simulink library "speedgoatlib"  (Simulink 7.6)
settings: Solver=ode45  StartTime=0.0  StopTime=10.0  RelTol=1e-3
undefined symbols (not defined in the file): m_XR17D15x, mmodemcontrol, standard
libraries: speedgoatlib x176, xpcseriallib x84, xpclib x4, simulink x4
(part 3 of 4)

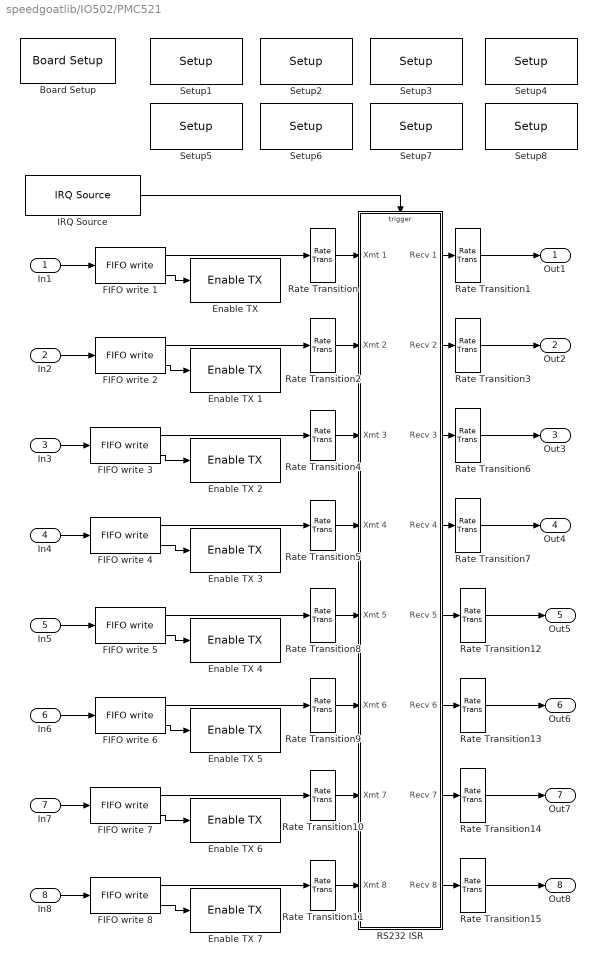
== system speedgoatlib/IO502/PMC521 ==
  In1 : Inport
  In2 : Inport  Port=2
  In3 : Inport  Port=3
  In4 : Inport  Port=4
  In5 : Inport  Port=5
  In6 : Inport  Port=6
  In7 : Inport  Port=7
  In8 : Inport  Port=8
  Board Setup : speedgoatlib/IO502/Acromag PMC521 Internal blocks/Board Setup  reffreq=14745600  irqnum=5  slot=brdslot
  "Enable TX " : speedgoatlib/IO502/Acromag PMC521 Internal blocks/Enable TX   port=1  slot=brdslot
  Enable TX 1 : speedgoatlib/IO502/Acromag PMC521 Internal blocks/Enable TX   port=2  slot=brdslot
  Enable TX 2 : speedgoatlib/IO502/Acromag PMC521 Internal blocks/Enable TX   port=3  slot=brdslot
  Enable TX 3 : speedgoatlib/IO502/Acromag PMC521 Internal blocks/Enable TX   port=4  slot=brdslot
  Enable TX 4 : speedgoatlib/IO502/Acromag PMC521 Internal blocks/Enable TX   port=5  slot=brdslot
  Enable TX 5 : speedgoatlib/IO502/Acromag PMC521 Internal blocks/Enable TX   port=6  slot=brdslot
  Enable TX 6 : speedgoatlib/IO502/Acromag PMC521 Internal blocks/Enable TX   port=7  slot=brdslot
  Enable TX 7 : speedgoatlib/IO502/Acromag PMC521 Internal blocks/Enable TX   port=8  slot=brdslot
  FIFO write 1 : xpcseriallib/FIFO write   size=1024  inputtype=8 bit uint null terminated  present=on  sampletime=-1  id=XMT channel 1, IRQ 5
  FIFO write 2 : xpcseriallib/FIFO write   size=1024  inputtype=8 bit uint null terminated  present=on  sampletime=-1  id=XMT channel 2, IRQ 5
  FIFO write 3 : xpcseriallib/FIFO write   size=1024  inputtype=8 bit uint null terminated  present=on  sampletime=-1  id=XMT channel 3, IRQ 5
  FIFO write 4 : xpcseriallib/FIFO write   size=1024  inputtype=8 bit uint null terminated  present=on  sampletime=-1  id=XMT channel 4, IRQ 5
  FIFO write 5 : xpcseriallib/FIFO write   size=1024  inputtype=8 bit uint null terminated  present=on  sampletime=-1  id=XMT channel 5, IRQ 5
  FIFO write 6 : xpcseriallib/FIFO write   size=1024  inputtype=8 bit uint null terminated  present=on  sampletime=-1  id=XMT channel 6, IRQ 5
  FIFO write 7 : xpcseriallib/FIFO write   size=1024  inputtype=8 bit uint null terminated  present=on  sampletime=-1  id=XMT channel 7, IRQ 5
  FIFO write 8 : xpcseriallib/FIFO write   size=1024  inputtype=8 bit uint null terminated  present=on  sampletime=-1  id=XMT channel 8, IRQ 5
  IRQ Source : xpclib/Asynchronous Event/IRQ Source  irqNo=5  preempt=off  b_type=None/Other  slot=brdslot
  RS232 ISR : Subsystem  TreatAsAtomicUnit=on  mask(RS232 ISR){slot=brdslot}
      mask help:
      | PMC521
      | Acromag
      | Interrupt Service Routine
      mask init:
      | subslot = slot;
      mask Display:
      | disp('PMC521\nAcromag\nISR');
      | port_label('input', 1, 'XMT1');
      | port_label('input', 2, 'XMT2');
      | port_label('input', 3, 'XMT3');
      | port_label('input', 4, 'XMT4');
      | port_label('input', 5, 'XMT5');
      | port_label('input', 6, 'XMT6');
      | port_label('input', 7, 'XMT7');
      | port_label('input', 8, 'XMT8');
      | port_label('output', 1, 'RCV1');
      | port_label('output', 2, 'RCV2');
      | port_label('output', 3, 'RCV3');
      | port_label('output', 4, 'RCV4');
      | port_label('output', 5, 'RCV5');
      | port_label('output', 6, 'RCV6');
      | port_label('output', 7, 'RCV7');
      | port_label('output', 8, 'RCV8');
  Rate Transition{,2,4..5,8..11} (8 alike) : RateTransition  Integrity=off  Deterministic=off
  Rate Transition{1,3,6..7,12..15} (8 alike) : RateTransition  Integrity=off  Deterministic=off  OutPortSampleTime=0
  Setup1 : speedgoatlib/IO502/Acromag PMC521 Internal blocks/Setup   port=1  standard=on  baudrate=115200  bauddivisor=1  mode8x=16x (standard)  prescale=off  width=8  nstop=1  parity=None  rlevel=1  ctsmode=none  xonoff=none  xon=17  xoff=19  rs485mode=off  rs485delay=0  slot=brdslot
  Setup2 : speedgoatlib/IO502/Acromag PMC521 Internal blocks/Setup   port=2  standard=on  baudrate=115200  bauddivisor=1  mode8x=16x (standard)  prescale=off  width=8  nstop=1  parity=None  rlevel=1  ctsmode=none  xonoff=none  xon=17  xoff=19  rs485mode=off  rs485delay=0  slot=brdslot
  Setup3 : speedgoatlib/IO502/Acromag PMC521 Internal blocks/Setup   port=3  standard=on  baudrate=115200  bauddivisor=1  mode8x=16x (standard)  prescale=off  width=8  nstop=1  parity=None  rlevel=half full (32)  ctsmode=none  xonoff=none  xon=17  xoff=19  rs485mode=off  rs485delay=0  slot=brdslot
  Setup4 : speedgoatlib/IO502/Acromag PMC521 Internal blocks/Setup   port=4  standard=on  baudrate=115200  bauddivisor=1  mode8x=16x (standard)  prescale=off  width=8  nstop=1  parity=None  rlevel=half full (32)  ctsmode=none  xonoff=none  xon=17  xoff=19  rs485mode=off  rs485delay=0  slot=brdslot
  Setup5 : speedgoatlib/IO502/Acromag PMC521 Internal blocks/Setup   port=5  standard=on  baudrate=115200  bauddivisor=1  mode8x=16x (standard)  prescale=off  width=8  nstop=1  parity=None  rlevel=1  ctsmode=none  xonoff=none  xon=17  xoff=19  rs485mode=off  rs485delay=0  slot=brdslot
  Setup6 : speedgoatlib/IO502/Acromag PMC521 Internal blocks/Setup   port=6  standard=on  baudrate=115200  bauddivisor=1  mode8x=16x (standard)  prescale=off  width=8  nstop=1  parity=None  rlevel=1  ctsmode=none  xonoff=none  xon=17  xoff=19  rs485mode=off  rs485delay=0  slot=brdslot
  Setup7 : speedgoatlib/IO502/Acromag PMC521 Internal blocks/Setup   port=7  standard=on  baudrate=115200  bauddivisor=1  mode8x=16x (standard)  prescale=off  width=8  nstop=1  parity=None  rlevel=1  ctsmode=none  xonoff=none  xon=17  xoff=19  rs485mode=off  rs485delay=0  slot=brdslot
  Setup8 : speedgoatlib/IO502/Acromag PMC521 Internal blocks/Setup   port=8  standard=on  baudrate=115200  bauddivisor=1  mode8x=16x (standard)  prescale=off  width=8  nstop=1  parity=None  rlevel=1  ctsmode=none  xonoff=none  xon=17  xoff=19  rs485mode=off  rs485delay=0  slot=brdslot
  Out1 : Outport
  Out2 : Outport  Port=2
  Out3 : Outport  Port=3
  Out4 : Outport  Port=4
  Out5 : Outport  Port=5
  Out6 : Outport  Port=6
  Out7 : Outport  Port=7
  Out8 : Outport  Port=8
  wires:
  RS232 ISR/8(Recv 8) -> Rate Transition15/1
  RS232 ISR/7(Recv 7) -> Rate Transition14/1
  RS232 ISR/6(Recv 6) -> Rate Transition13/1
  RS232 ISR/5(Recv 5) -> Rate Transition12/1
  Rate Transition13/1 -> Out6/1
  Rate Transition12/1 -> Out5/1
  Rate Transition14/1 -> Out7/1
  Rate Transition15/1 -> Out8/1
  FIFO write 6/2 -> Enable TX 5/1
  In6/1 -> FIFO write 6/1
  FIFO write 6/1 -> Rate Transition9/1
  In5/1 -> FIFO write 5/1
  FIFO write 5/1 -> Rate Transition8/1
  FIFO write 5/2 -> Enable TX 4/1
  Rate Transition9/1 -> RS232 ISR/6(Xmt 6)
  Rate Transition8/1 -> RS232 ISR/5(Xmt 5)
  FIFO write 7/2 -> Enable TX 6/1
  In7/1 -> FIFO write 7/1
  FIFO write 7/1 -> Rate Transition10/1
  FIFO write 8/2 -> Enable TX 7/1
  In8/1 -> FIFO write 8/1
  FIFO write 8/1 -> Rate Transition11/1
  Rate Transition10/1 -> RS232 ISR/7(Xmt 7)
  Rate Transition11/1 -> RS232 ISR/8(Xmt 8)
  FIFO write 2/2 -> Enable TX 1/1
  In2/1 -> FIFO write 2/1
  FIFO write 2/1 -> Rate Transition2/1
  In1/1 -> FIFO write 1/1
  FIFO write 1/1 -> Rate Transition/1
  RS232 ISR/2(Recv 2) -> Rate Transition3/1
  RS232 ISR/1(Recv 1) -> Rate Transition1/1
  IRQ Source/1 -> RS232 ISR/Trigger
  FIFO write 1/2 -> "Enable TX "/1
  Rate Transition2/1 -> RS232 ISR/2(Xmt 2)
  Rate Transition/1 -> RS232 ISR/1(Xmt 1)
  Rate Transition3/1 -> Out2/1
  Rate Transition1/1 -> Out1/1
  FIFO write 3/2 -> Enable TX 2/1
  In3/1 -> FIFO write 3/1
  FIFO write 3/1 -> Rate Transition4/1
  FIFO write 4/2 -> Enable TX 3/1
  In4/1 -> FIFO write 4/1
  FIFO write 4/1 -> Rate Transition5/1
  Rate Transition4/1 -> RS232 ISR/3(Xmt 3)
  Rate Transition5/1 -> RS232 ISR/4(Xmt 4)
  Rate Transition6/1 -> Out3/1
  Rate Transition7/1 -> Out4/1
  RS232 ISR/3(Recv 3) -> Rate Transition6/1
  RS232 ISR/4(Recv 4) -> Rate Transition7/1

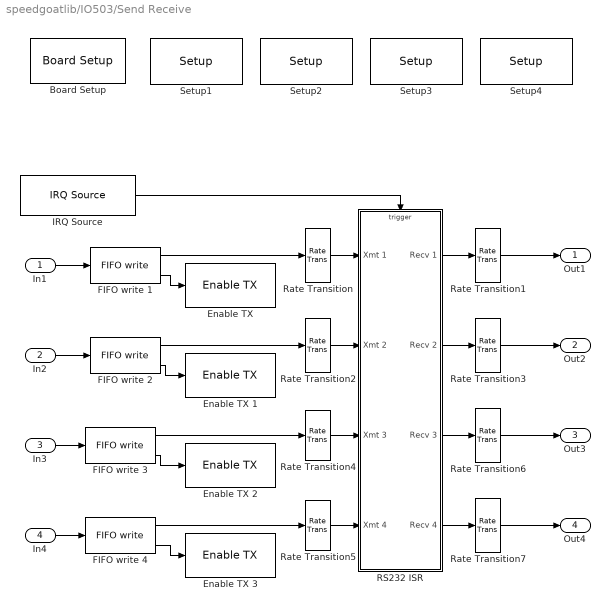
== system speedgoatlib/IO503/Send Receive ==
  In1 : Inport
  In2 : Inport  Port=2
  In3 : Inport  Port=3
  In4 : Inport  Port=4
  Board Setup : speedgoatlib/IO503/Speedgoat IO503 Internal blocks/Board Setup  irqnum=5  slot=brdslot
  "Enable TX " : speedgoatlib/IO503/Speedgoat IO503 Internal blocks/Enable TX  port=1  slot=brdslot
  Enable TX 1 : speedgoatlib/IO503/Speedgoat IO503 Internal blocks/Enable TX  port=2  slot=brdslot
  Enable TX 2 : speedgoatlib/IO503/Speedgoat IO503 Internal blocks/Enable TX  port=3  slot=brdslot
  Enable TX 3 : speedgoatlib/IO503/Speedgoat IO503 Internal blocks/Enable TX  port=4  slot=brdslot
  FIFO write 1 : xpcseriallib/FIFO write   size=1024  inputtype=8 bit uint null terminated  present=on  sampletime=-1  id=XMT channel 1, IRQ 5
  FIFO write 2 : xpcseriallib/FIFO write   size=1024  inputtype=8 bit uint null terminated  present=on  sampletime=-1  id=XMT channel 2, IRQ 5
  FIFO write 3 : xpcseriallib/FIFO write   size=1024  inputtype=8 bit uint null terminated  present=on  sampletime=-1  id=XMT channel 3, IRQ 5
  FIFO write 4 : xpcseriallib/FIFO write   size=1024  inputtype=8 bit uint null terminated  present=on  sampletime=-1  id=XMT channel 4, IRQ 5
  IRQ Source : xpclib/Asynchronous Event/IRQ Source  irqNo=5  preempt=off  b_type=None/Other  slot=brdslot
  RS232 ISR : Subsystem  TreatAsAtomicUnit=on  mask(RS232 ISR){slot=brdslot}
      mask help:
      | Speedgoat
      | IO503
      | Interrupt Service Routine
      mask init:
      | subslot = slot;
      mask Display:
      | disp('Speedgoat\nIO503\nISR');
      | port_label('input', 1, 'XMT1');
      | port_label('input', 2, 'XMT2');
      | port_label('input', 3, 'XMT3');
      | port_label('input', 4, 'XMT4');
      | port_label('output', 1, 'RCV1');
      | port_label('output', 2, 'RCV2');
      | port_label('output', 3, 'RCV3');
      | port_label('output', 4, 'RCV4');
  Rate Transition{,2,4..5} (4 alike) : RateTransition  Integrity=off  Deterministic=off
  Rate Transition{1,3,6..7} (4 alike) : RateTransition  Integrity=off  Deterministic=off  OutPortSampleTime=0
  Setup1 : speedgoatlib/IO503/Speedgoat IO503 Internal blocks/Setup  port=1  transceiver=RS232 (max 921.6kb/s)  standard=on  baudrate=115200  bauddivisor=1  mode8x=16x (standard)  prescale=off  width=8  nstop=1  parity=None  rlevel=1  ctsmode=none  xonoff=none  xon=17  xoff=19  rs485mode=off  rs485delay=0  slot=brdslot
  Setup2 : speedgoatlib/IO503/Speedgoat IO503 Internal blocks/Setup  port=2  transceiver=RS232 (max 921.6kb/s)  standard=on  baudrate=115200  bauddivisor=1  mode8x=16x (standard)  prescale=off  width=8  nstop=1  parity=None  rlevel=1  ctsmode=none  xonoff=none  xon=17  xoff=19  rs485mode=off  rs485delay=0  slot=brdslot
  Setup3 : speedgoatlib/IO503/Speedgoat IO503 Internal blocks/Setup  port=3  transceiver=RS232 (max 921.6kb/s)  standard=on  baudrate=115200  bauddivisor=1  mode8x=16x (standard)  prescale=off  width=8  nstop=1  parity=None  rlevel=half full (32)  ctsmode=none  xonoff=none  xon=17  xoff=19  rs485mode=off  rs485delay=0  slot=brdslot
  Setup4 : speedgoatlib/IO503/Speedgoat IO503 Internal blocks/Setup  port=4  transceiver=RS232 (max 921.6kb/s)  standard=on  baudrate=115200  bauddivisor=1  mode8x=16x (standard)  prescale=off  width=8  nstop=1  parity=None  rlevel=half full (32)  ctsmode=none  xonoff=none  xon=17  xoff=19  rs485mode=off  rs485delay=0  slot=brdslot
  Out1 : Outport
  Out2 : Outport  Port=2
  Out3 : Outport  Port=3
  Out4 : Outport  Port=4
  wires:
  FIFO write 2/2 -> Enable TX 1/1
  In2/1 -> FIFO write 2/1
  FIFO write 2/1 -> Rate Transition2/1
  In1/1 -> FIFO write 1/1
  FIFO write 1/1 -> Rate Transition/1
  RS232 ISR/2(Recv 2) -> Rate Transition3/1
  RS232 ISR/1(Recv 1) -> Rate Transition1/1
  IRQ Source/1 -> RS232 ISR/Trigger
  FIFO write 1/2 -> "Enable TX "/1
  Rate Transition2/1 -> RS232 ISR/2(Xmt 2)
  Rate Transition/1 -> RS232 ISR/1(Xmt 1)
  Rate Transition3/1 -> Out2/1
  Rate Transition1/1 -> Out1/1
  FIFO write 3/2 -> Enable TX 2/1
  In3/1 -> FIFO write 3/1
  FIFO write 3/1 -> Rate Transition4/1
  FIFO write 4/2 -> Enable TX 3/1
  In4/1 -> FIFO write 4/1
  FIFO write 4/1 -> Rate Transition5/1
  Rate Transition4/1 -> RS232 ISR/3(Xmt 3)
  Rate Transition5/1 -> RS232 ISR/4(Xmt 4)
  Rate Transition6/1 -> Out3/1
  Rate Transition7/1 -> Out4/1
  RS232 ISR/3(Recv 3) -> Rate Transition6/1
  RS232 ISR/4(Recv 4) -> Rate Transition7/1

== system speedgoatlib/IO503/Speedgoat IO503 Internal blocks ==
  Board Setup : S-Function  FunctionName=board_setup_tews_XR17D15x  Parameters=slot, irqnum+2, 102  EnableBusSupport=off  mask(board_setup_XR17D15x){irqnum=5, slot=-1}
      mask prompts: irqnum "IRQ Line Number"; slot "PCI slot: (-1 for autosearch)"
      mask help:
      | Speedgoat
      | IO503
      | Board Setup
      mask Help: helpview(fullfile(docroot, 'mapfiles', 'xpc.map'), 'Commtech_422335_IntChk')
      mask StyleString: popup(3|4|5|6|7|8|9|10|11|12|13|14|15),edit
      mask Display: disp('Speedgoat\nIO503\nBoard Setup');
  Enable TX : S-Function  FunctionName=tx_int_enable_XR17D15x  Parameters=slot, port, 102  EnableBusSupport=off  mask(tx_int_enable_XR17D15x){port=1, slot=-1}
      mask prompts: slot "PCI slot: (-1 for autosearch)"
      mask help:
      | Speedgoat
      | IO503
      | Enable TX Interrupt
      mask Help: helpview(fullfile(docroot, 'mapfiles', 'xpc.map'), 'FC422335_Enable_Int')
      mask StyleString: popup(1|2|3|4),edit
      mask Display:
      | disp('Speedgoat\nIO503\nEnable TX int');
      | port_label('input', 1, 'E');
  Int Source Filter : S-Function  FunctionName=int_source_filter_XR17D15x  Parameters=port, 102, value  EnableBusSupport=off  mask(int_source_filter_XR17D15x){port=1, value=Receive data}
      mask prompts: value "Filter value:"
      mask help:
      | Speedgoat
      | IO503
      | Interrupt Source Filter
      mask Help: helpview(fullfile(docroot, 'mapfiles', 'xpc.map'), 'FC422335_Filter_Ints')
      mask StyleString: popup(1|2|3|4),popup(Receive data|Transmitter empty|Modem status change)
      mask Display:
      | disp('Speedgoat\nIO503\nInt Source Filter');
      | port_label('input', 1, 'S' );
      | port_label('output', 1, 'E' );
  Read HW FIFO : S-Function  FunctionName=read_hw_fifo_XR17D15x  Parameters=slot, port, 102, flush  EnableBusSupport=off  mask(read_hw_fifo_XR17D15x){port=1, flush=on, slot=-1}
      mask prompts: flush "Flush HW FIFO on startup"; slot "PCI slot: (-1 for autosearch)"
      mask help:
      | Speedgoat
      | IO503
      | Read Hardware FIFO
      mask Help: helpview(fullfile(docroot, 'mapfiles', 'xpc.map'), 'FC422335_Read_HW')
      mask StyleString: popup(1|2|3|4),checkbox,edit
      mask Display:
      | disp('Speedgoat\nIO503\nRead HW FIFO');
      | port_label('input', 1, 'E');
      | port_label('output', 1, 'D');
  Read Int Status : S-Function  FunctionName=read_int_status_XR17D15x  Parameters=slot, 102  EnableBusSupport=off  mask(read_int_status_XR17D15x){slot=-1}
      mask prompts: slot "PCI slot: (-1 for autosearch)"
      mask help:
      | Speedgoat
      | IO503
      | Read Interrupt Status
      mask Help: helpview(fullfile(docroot, 'mapfiles', 'xpc.map'), 'Commtech_422335_Interrupt_Query')
      mask Display:
      | disp('Speedgoat\nIO503\nRead Int Status');
      | port_label('output', 1, 'S' );
  Setup : S-Function  FunctionName=setup_tews_XR17D15x  Parameters=slot, 102, port, standard, baudrate, bauddivisor, mode8x, prescale, width, nstop, parity, rlevel, ctsmode, xonoff, xon, xoff, rs485mode, rs485delay, transceiver  EnableBusSupport=off  mask(setup_XR17D15x){port=1, transceiver=RS232 (max 921.6kb/s), standard=on, baudrate=115200, bauddivisor=1, mode8x=16x (standard), prescale=off, width=8, nstop=1, parity=None, rlevel=1, ctsmode=none, xonoff=none, xon=17, xoff=19, rs485mode=off, rs485delay=0, slot=-1}
      mask prompts: transceiver "Transceiver setup:"; standard "Use standard baud rates (16x, no prescaling)"; baudrate "Standard baud rate:"; bauddivisor "Baud rate divisor (non-standard baud rates):"; mode8x "Sampling rate (non-standard baud rates):"; prescale "Prescale by 4 (non-standard baud rates)"; width "Number of data bits:"; nstop "Number of stop bits:"; rlevel "Receive trigger level:"; ctsmode "Hardware handshake:"; xonoff "Software handshake:"; xon "XON character:"; xoff "XOFF character:"; rs485mode "RS485 auto turnaround"; rs485delay "RS485 turnaround delay:"; slot "PCI slot: (-1 for autosearch)"
      mask help:
      | Speedgoat
      | IO503
      | Setup
      mask Help: helpview(fullfile(docroot, 'mapfiles', 'xpc.map'), 'FC422335_Setup')
      mask StyleString: edit,popup(RS232 (max 921.6kb/s)|RS422|RS422 multidrop|RS485 full-duplex|RS485 half-duplex),checkbox,popup(2764800|1382400|921600|460800|230400|115200|57600|38400|19200|9600|4800|2400|1200|600|400),edit,popup(8x|16x (standard)),checkbox,popup(5|6|7|8),popup(1|2),popup(None|Even|Odd|Mark|Space),popup(1|quarter full (16)|half full (32)|almost full (56)),popup(RTS/CTS|DTR/DSR|none),popup(XON/XOFF|none),edit,edit,checkbox,edit,edit
      mask Display: disp('Speedgoat\nIO503\nSetup');
  Write HW FIFO : S-Function  FunctionName=write_hw_fifo_XR17D15x  Parameters=slot, port, 102  EnableBusSupport=off  mask(write_hw_fifo_XR17D15x){port=1, slot=-1}
      mask prompts: slot "PCI slot: (-1 for autosearch)"
      mask help:
      | Speedgoat
      | IO503
      | Write Hardware FIFO
      mask Help: helpview(fullfile(docroot, 'mapfiles', 'xpc.map'), 'FC422335_Write_HW')
      mask StyleString: popup(1|2|3|4),edit
      mask Display:
      | disp('Speedgoat\nIO503\nWrite HW FIFO');
      | port_label('input', 1, 'D');
      | port_label('input', 2, 'E');

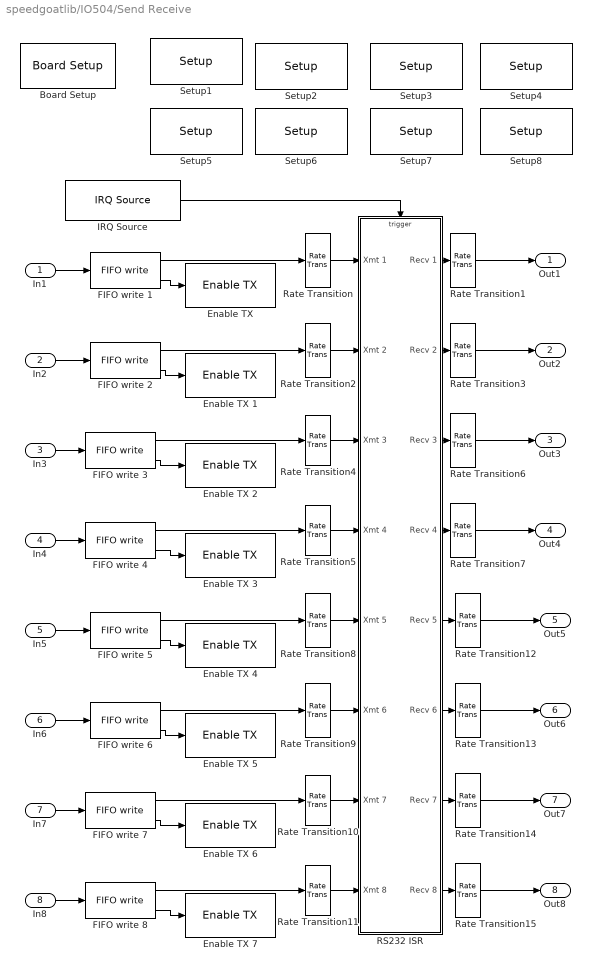
== system speedgoatlib/IO504/Send Receive ==
  In1 : Inport
  In2 : Inport  Port=2
  In3 : Inport  Port=3
  In4 : Inport  Port=4
  In5 : Inport  Port=5
  In6 : Inport  Port=6
  In7 : Inport  Port=7
  In8 : Inport  Port=8
  Board Setup : speedgoatlib/IO504/Speedgoat IO504 Internal blocks/Board Setup  irqnum=5  slot=brdslot
  "Enable TX " : speedgoatlib/IO504/Speedgoat IO504 Internal blocks/Enable TX  port=1  slot=brdslot
  Enable TX 1 : speedgoatlib/IO504/Speedgoat IO504 Internal blocks/Enable TX  port=2  slot=brdslot
  Enable TX 2 : speedgoatlib/IO504/Speedgoat IO504 Internal blocks/Enable TX  port=3  slot=brdslot
  Enable TX 3 : speedgoatlib/IO504/Speedgoat IO504 Internal blocks/Enable TX  port=4  slot=brdslot
  Enable TX 4 : speedgoatlib/IO504/Speedgoat IO504 Internal blocks/Enable TX  port=5  slot=brdslot
  Enable TX 5 : speedgoatlib/IO504/Speedgoat IO504 Internal blocks/Enable TX  port=6  slot=brdslot
  Enable TX 6 : speedgoatlib/IO504/Speedgoat IO504 Internal blocks/Enable TX  port=7  slot=brdslot
  Enable TX 7 : speedgoatlib/IO504/Speedgoat IO504 Internal blocks/Enable TX  port=8  slot=brdslot
  FIFO write 1 : xpcseriallib/FIFO write   size=1024  inputtype=8 bit uint null terminated  present=on  sampletime=-1  id=XMT channel 1, IRQ 5
  FIFO write 2 : xpcseriallib/FIFO write   size=1024  inputtype=8 bit uint null terminated  present=on  sampletime=-1  id=XMT channel 2, IRQ 5
  FIFO write 3 : xpcseriallib/FIFO write   size=1024  inputtype=8 bit uint null terminated  present=on  sampletime=-1  id=XMT channel 3, IRQ 5
  FIFO write 4 : xpcseriallib/FIFO write   size=1024  inputtype=8 bit uint null terminated  present=on  sampletime=-1  id=XMT channel 4, IRQ 5
  FIFO write 5 : xpcseriallib/FIFO write   size=1024  inputtype=8 bit uint null terminated  present=on  sampletime=-1  id=XMT channel 5, IRQ 5
  FIFO write 6 : xpcseriallib/FIFO write   size=1024  inputtype=8 bit uint null terminated  present=on  sampletime=-1  id=XMT channel 6, IRQ 5
  FIFO write 7 : xpcseriallib/FIFO write   size=1024  inputtype=8 bit uint null terminated  present=on  sampletime=-1  id=XMT channel 7, IRQ 5
  FIFO write 8 : xpcseriallib/FIFO write   size=1024  inputtype=8 bit uint null terminated  present=on  sampletime=-1  id=XMT channel 8, IRQ 5
  IRQ Source : xpclib/Asynchronous Event/IRQ Source  irqNo=5  preempt=off  b_type=None/Other  slot=brdslot
  RS232 ISR : Subsystem  TreatAsAtomicUnit=on  mask(RS232 ISR){slot=brdslot}
      mask help:
      | PMC521
      | Acromag
      | Interrupt Service Routine
      mask init:
      | subslot = slot;
      mask Display:
      | disp('Speedgoat\nIO504\nISR');
      | port_label('input', 1, 'XMT1');
      | port_label('input', 2, 'XMT2');
      | port_label('input', 3, 'XMT3');
      | port_label('input', 4, 'XMT4');
      | port_label('input', 5, 'XMT5');
      | port_label('input', 6, 'XMT6');
      | port_label('input', 7, 'XMT7');
      | port_label('input', 8, 'XMT8');
      | port_label('output', 1, 'RCV1');
      | port_label('output', 2, 'RCV2');
      | port_label('output', 3, 'RCV3');
      | port_label('output', 4, 'RCV4');
      | port_label('output', 5, 'RCV5');
      | port_label('output', 6, 'RCV6');
      | port_label('output', 7, 'RCV7');
      | port_label('output', 8, 'RCV8');
  Rate Transition{,2,4..5,8..11} (8 alike) : RateTransition  Integrity=off  Deterministic=off
  Rate Transition{1,3,6..7,12..15} (8 alike) : RateTransition  Integrity=off  Deterministic=off  OutPortSampleTime=0
  Setup1 : speedgoatlib/IO504/Speedgoat IO504 Internal blocks/Setup  port=1  transceiver=RS232 (max 921.6kb/s)  standard=on  baudrate=115200  bauddivisor=1  mode8x=16x (standard)  prescale=off  width=8  nstop=1  parity=None  rlevel=1  ctsmode=none  xonoff=none  xon=17  xoff=19  rs485mode=off  rs485delay=0  slot=brdslot
  Setup2 : speedgoatlib/IO504/Speedgoat IO504 Internal blocks/Setup  port=2  transceiver=RS232 (max 921.6kb/s)  standard=on  baudrate=115200  bauddivisor=1  mode8x=16x (standard)  prescale=off  width=8  nstop=1  parity=None  rlevel=1  ctsmode=none  xonoff=none  xon=17  xoff=19  rs485mode=off  rs485delay=0  slot=brdslot
  Setup3 : speedgoatlib/IO504/Speedgoat IO504 Internal blocks/Setup  port=3  transceiver=RS232 (max 921.6kb/s)  standard=on  baudrate=115200  bauddivisor=1  mode8x=16x (standard)  prescale=off  width=8  nstop=1  parity=None  rlevel=half full (32)  ctsmode=none  xonoff=none  xon=17  xoff=19  rs485mode=off  rs485delay=0  slot=brdslot
  Setup4 : speedgoatlib/IO504/Speedgoat IO504 Internal blocks/Setup  port=4  transceiver=RS232 (max 921.6kb/s)  standard=on  baudrate=115200  bauddivisor=1  mode8x=16x (standard)  prescale=off  width=8  nstop=1  parity=None  rlevel=half full (32)  ctsmode=none  xonoff=none  xon=17  xoff=19  rs485mode=off  rs485delay=0  slot=brdslot
  Setup5 : speedgoatlib/IO504/Speedgoat IO504 Internal blocks/Setup  port=5  transceiver=RS232 (max 921.6kb/s)  standard=on  baudrate=115200  bauddivisor=1  mode8x=16x (standard)  prescale=off  width=8  nstop=1  parity=None  rlevel=1  ctsmode=none  xonoff=none  xon=17  xoff=19  rs485mode=off  rs485delay=0  slot=brdslot
  Setup6 : speedgoatlib/IO504/Speedgoat IO504 Internal blocks/Setup  port=6  transceiver=RS232 (max 921.6kb/s)  standard=on  baudrate=115200  bauddivisor=1  mode8x=16x (standard)  prescale=off  width=8  nstop=1  parity=None  rlevel=1  ctsmode=none  xonoff=none  xon=17  xoff=19  rs485mode=off  rs485delay=0  slot=brdslot
  Setup7 : speedgoatlib/IO504/Speedgoat IO504 Internal blocks/Setup  port=7  transceiver=RS232 (max 921.6kb/s)  standard=on  baudrate=115200  bauddivisor=1  mode8x=16x (standard)  prescale=off  width=8  nstop=1  parity=None  rlevel=1  ctsmode=none  xonoff=none  xon=17  xoff=19  rs485mode=off  rs485delay=0  slot=brdslot
  Setup8 : speedgoatlib/IO504/Speedgoat IO504 Internal blocks/Setup  port=8  transceiver=RS232 (max 921.6kb/s)  standard=on  baudrate=115200  bauddivisor=1  mode8x=16x (standard)  prescale=off  width=8  nstop=1  parity=None  rlevel=1  ctsmode=none  xonoff=none  xon=17  xoff=19  rs485mode=off  rs485delay=0  slot=brdslot
  Out1 : Outport
  Out2 : Outport  Port=2
  Out3 : Outport  Port=3
  Out4 : Outport  Port=4
  Out5 : Outport  Port=5
  Out6 : Outport  Port=6
  Out7 : Outport  Port=7
  Out8 : Outport  Port=8
  wires:
  RS232 ISR/4(Recv 4) -> Rate Transition7/1
  RS232 ISR/3(Recv 3) -> Rate Transition6/1
  Rate Transition7/1 -> Out4/1
  Rate Transition6/1 -> Out3/1
  Rate Transition5/1 -> RS232 ISR/4(Xmt 4)
  Rate Transition4/1 -> RS232 ISR/3(Xmt 3)
  FIFO write 4/1 -> Rate Transition5/1
  In4/1 -> FIFO write 4/1
  FIFO write 4/2 -> Enable TX 3/1
  FIFO write 3/1 -> Rate Transition4/1
  In3/1 -> FIFO write 3/1
  FIFO write 3/2 -> Enable TX 2/1
  Rate Transition1/1 -> Out1/1
  Rate Transition3/1 -> Out2/1
  Rate Transition/1 -> RS232 ISR/1(Xmt 1)
  Rate Transition2/1 -> RS232 ISR/2(Xmt 2)
  FIFO write 1/2 -> "Enable TX "/1
  IRQ Source/1 -> RS232 ISR/Trigger
  RS232 ISR/1(Recv 1) -> Rate Transition1/1
  RS232 ISR/2(Recv 2) -> Rate Transition3/1
  FIFO write 1/1 -> Rate Transition/1
  In1/1 -> FIFO write 1/1
  FIFO write 2/1 -> Rate Transition2/1
  In2/1 -> FIFO write 2/1
  FIFO write 2/2 -> Enable TX 1/1
  Rate Transition11/1 -> RS232 ISR/8(Xmt 8)
  Rate Transition10/1 -> RS232 ISR/7(Xmt 7)
  FIFO write 8/1 -> Rate Transition11/1
  In8/1 -> FIFO write 8/1
  FIFO write 8/2 -> Enable TX 7/1
  FIFO write 7/1 -> Rate Transition10/1
  In7/1 -> FIFO write 7/1
  FIFO write 7/2 -> Enable TX 6/1
  Rate Transition8/1 -> RS232 ISR/5(Xmt 5)
  Rate Transition9/1 -> RS232 ISR/6(Xmt 6)
  FIFO write 5/2 -> Enable TX 4/1
  FIFO write 5/1 -> Rate Transition8/1
  In5/1 -> FIFO write 5/1
  FIFO write 6/1 -> Rate Transition9/1
  In6/1 -> FIFO write 6/1
  FIFO write 6/2 -> Enable TX 5/1
  Rate Transition15/1 -> Out8/1
  Rate Transition14/1 -> Out7/1
  Rate Transition12/1 -> Out5/1
  Rate Transition13/1 -> Out6/1
  RS232 ISR/5(Recv 5) -> Rate Transition12/1
  RS232 ISR/6(Recv 6) -> Rate Transition13/1
  RS232 ISR/7(Recv 7) -> Rate Transition14/1
  RS232 ISR/8(Recv 8) -> Rate Transition15/1

== system speedgoatlib/IO504/Speedgoat IO504 Internal blocks ==
  Board Setup : S-Function  FunctionName=board_setup_tews_XR17D15x  Parameters=slot, irqnum+2 103  EnableBusSupport=off  mask(board_setup_XR17D15x){irqnum=5, slot=-1}
      mask prompts: irqnum "IRQ Line Number"; slot "PCI slot: (-1 for autosearch)"
      mask help:
      | Speedgoat
      | IO504
      | Board Setup
      mask Help: helpview(fullfile(docroot, 'mapfiles', 'xpc.map'), 'Commtech_422335_IntChk')
      mask StyleString: popup(3|4|5|6|7|8|9|10|11|12|13|14|15),edit
      mask Display: disp('Speedgoat\nIO504\nBoard Setup');
  Enable TX : S-Function  FunctionName=tx_int_enable_XR17D15x  Parameters=slot, port, 103  EnableBusSupport=off  mask(tx_int_enable_XR17D15x){port=1, slot=-1}
      mask prompts: slot "PCI slot: (-1 for autosearch)"
      mask help:
      | Speedgoat
      | IO504
      | Enable TX Interrupt
      mask Help: helpview(fullfile(docroot, 'mapfiles', 'xpc.map'), 'FC422335_Enable_Int')
      mask StyleString: popup(1|2|3|4|5|6|7|8),edit
      mask Display:
      | disp('Speedgoat\nIO504\nEnable TX int');
      | port_label('input', 1, 'E');
  Int Source Filter : S-Function  FunctionName=int_source_filter_XR17D15x  Parameters=port, 103, value  EnableBusSupport=off  mask(int_source_filter_XR17D15x){port=1, value=Receive data}
      mask prompts: value "Filter value:"
      mask help:
      | Speedgoat
      | IO504
      | Interrupt Source Filter
      mask Help: helpview(fullfile(docroot, 'mapfiles', 'xpc.map'), 'FC422335_Filter_Ints')
      mask StyleString: popup(1|2|3|4|5|6|7|8),popup(Receive data|Transmitter empty|Modem status change)
      mask Display:
      | disp('Speedgoat\nIO504\nInt Source Filter');
      | port_label('input', 1, 'S' );
      | port_label('output', 1, 'E' );
  Read HW FIFO : S-Function  FunctionName=read_hw_fifo_XR17D15x  Parameters=slot, port, 103, flush  EnableBusSupport=off  mask(read_hw_fifo_XR17D15x){port=1, flush=on, slot=-1}
      mask prompts: flush "Flush HW FIFO on startup"; slot "PCI slot: (-1 for autosearch)"
      mask help:
      | Speedgoat
      | IO504
      | Read Hardware FIFO
      mask Help: helpview(fullfile(docroot, 'mapfiles', 'xpc.map'), 'FC422335_Read_HW')
      mask StyleString: popup(1|2|3|4|5|6|7|8),checkbox,edit
      mask Display:
      | disp('Speedgoat\nIO504\nRead HW FIFO');
      | port_label('input', 1, 'E');
      | port_label('output', 1, 'D');
  Read Int Status : S-Function  FunctionName=read_int_status_XR17D15x  Parameters=slot, 103  EnableBusSupport=off  mask(read_int_status_XR17D15x){slot=-1}
      mask prompts: slot "PCI slot: (-1 for autosearch)"
      mask help:
      | TPMC465
      | TEWS
      | Read Interrupt Status
      mask Help: helpview(fullfile(docroot, 'mapfiles', 'xpc.map'), 'Commtech_422335_Interrupt_Query')
      mask Display:
      | disp('Speedgoat\nIO504\nRead Int Status');
      | port_label('output', 1, 'S' );
  Setup : S-Function  FunctionName=setup_tews_XR17D15x  Parameters=slot, 103, port, standard, baudrate, bauddivisor, mode8x, prescale, width, nstop, parity, rlevel, ctsmode, xonoff, xon, xoff, rs485mode, rs485delay, transceiver  EnableBusSupport=off  mask(setup_XR17D15x){port=1, transceiver=RS232 (max 921.6kb/s), standard=on, baudrate=115200, bauddivisor=1, mode8x=16x (standard), prescale=off, width=8, nstop=1, parity=None, rlevel=1, ctsmode=none, xonoff=none, xon=17, xoff=19, rs485mode=off, rs485delay=0, slot=-1}
      mask prompts: transceiver "Transceiver setup:"; standard "Use standard baud rates (16x, no prescaling)"; baudrate "Standard baud rate:"; bauddivisor "Baud rate divisor (non-standard baud rates):"; mode8x "Sampling rate (non-standard baud rates):"; prescale "Prescale by 4 (non-standard baud rates)"; width "Number of data bits:"; nstop "Number of stop bits:"; rlevel "Receive trigger level:"; ctsmode "Hardware handshake:"; xonoff "Software handshake:"; xon "XON character:"; xoff "XOFF character:"; rs485mode "RS485 auto turnaround"; rs485delay "RS485 turnaround delay:"; slot "PCI slot: (-1 for autosearch)"
      mask help:
      | TPMC465
      | TEWS
      | Setup
      mask Help: helpview(fullfile(docroot, 'mapfiles', 'xpc.map'), 'FC422335_Setup')
      mask StyleString: edit,popup(RS232 (max 921.6kb/s)|RS422|RS422 multidrop|RS485 full-duplex|RS485 half-duplex),checkbox,popup(2764800|1382400|921600|460800|230400|115200|57600|38400|19200|9600|4800|2400|1200|600|400),edit,popup(8x|16x (standard)),checkbox,popup(5|6|7|8),popup(1|2),popup(None|Even|Odd|Mark|Space),popup(1|quarter full (16)|half full (32)|almost full (56)),popup(RTS/CTS|DTR/DSR|none),popup(XON/XOFF|none),edit,edit,checkbox,edit,edit
      mask Display: disp('Speedgoat\nIO504\nSetup');
  Write HW FIFO : S-Function  FunctionName=write_hw_fifo_XR17D15x  Parameters=slot, port, 103  EnableBusSupport=off  mask(write_hw_fifo_XR17D15x){port=1, slot=-1}
      mask prompts: slot "PCI slot: (-1 for autosearch)"
      mask help:
      | Speedgoat
      | IO504
      | Write Hardware FIFO
      mask Help: helpview(fullfile(docroot, 'mapfiles', 'xpc.map'), 'FC422335_Write_HW')
      mask StyleString: popup(1|2|3|4|5|6|7|8),edit
      mask Display:
      | disp('Speedgoat\nIO504\nWrite HW FIFO');
      | port_label('input', 1, 'D');
      | port_label('input', 2, 'E');

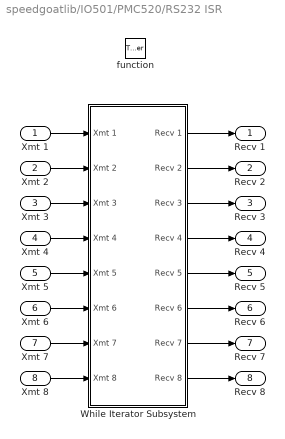
== system speedgoatlib/IO501/PMC520/RS232 ISR ==
  Xmt 1 : Inport
  Xmt 2 : Inport  Port=2
  Xmt 3 : Inport  Port=3
  Xmt 4 : Inport  Port=4
  Xmt 5 : Inport  Port=5
  Xmt 6 : Inport  Port=6
  Xmt 7 : Inport  Port=7
  Xmt 8 : Inport  Port=8
  function : TriggerPort  TriggerType=function-call
  While Iterator Subsystem : Subsystem  TreatAsAtomicUnit=on
  Recv 1 : Outport
  Recv 2 : Outport  Port=2
  Recv 3 : Outport  Port=3
  Recv 4 : Outport  Port=4
  Recv 5 : Outport  Port=5
  Recv 6 : Outport  Port=6
  Recv 7 : Outport  Port=7
  Recv 8 : Outport  Port=8
  wires:
  While Iterator Subsystem/4(Recv 4) -> Recv 4/1
  While Iterator Subsystem/3(Recv 3) -> Recv 3/1
  Xmt 4/1 -> While Iterator Subsystem/4(Xmt 4)
  Xmt 3/1 -> While Iterator Subsystem/3(Xmt 3)
  While Iterator Subsystem/2(Recv 2) -> Recv 2/1
  While Iterator Subsystem/1(Recv 1) -> Recv 1/1
  Xmt 2/1 -> While Iterator Subsystem/2(Xmt 2)
  Xmt 1/1 -> While Iterator Subsystem/1(Xmt 1)
  Xmt 8/1 -> While Iterator Subsystem/8(Xmt 8)
  Xmt 7/1 -> While Iterator Subsystem/7(Xmt 7)
  Xmt 6/1 -> While Iterator Subsystem/6(Xmt 6)
  Xmt 5/1 -> While Iterator Subsystem/5(Xmt 5)
  While Iterator Subsystem/8(Recv 8) -> Recv 8/1
  While Iterator Subsystem/7(Recv 7) -> Recv 7/1
  While Iterator Subsystem/6(Recv 6) -> Recv 6/1
  While Iterator Subsystem/5(Recv 5) -> Recv 5/1

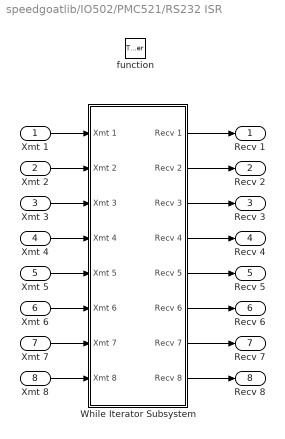
== system speedgoatlib/IO502/PMC521/RS232 ISR ==
  Xmt 1 : Inport
  Xmt 2 : Inport  Port=2
  Xmt 3 : Inport  Port=3
  Xmt 4 : Inport  Port=4
  Xmt 5 : Inport  Port=5
  Xmt 6 : Inport  Port=6
  Xmt 7 : Inport  Port=7
  Xmt 8 : Inport  Port=8
  function : TriggerPort  TriggerType=function-call
  While Iterator Subsystem : Subsystem  TreatAsAtomicUnit=on
  Recv 1 : Outport
  Recv 2 : Outport  Port=2
  Recv 3 : Outport  Port=3
  Recv 4 : Outport  Port=4
  Recv 5 : Outport  Port=5
  Recv 6 : Outport  Port=6
  Recv 7 : Outport  Port=7
  Recv 8 : Outport  Port=8
  wires:
  While Iterator Subsystem/5(Recv 5) -> Recv 5/1
  While Iterator Subsystem/6(Recv 6) -> Recv 6/1
  While Iterator Subsystem/7(Recv 7) -> Recv 7/1
  While Iterator Subsystem/8(Recv 8) -> Recv 8/1
  Xmt 5/1 -> While Iterator Subsystem/5(Xmt 5)
  Xmt 6/1 -> While Iterator Subsystem/6(Xmt 6)
  Xmt 7/1 -> While Iterator Subsystem/7(Xmt 7)
  Xmt 8/1 -> While Iterator Subsystem/8(Xmt 8)
  Xmt 1/1 -> While Iterator Subsystem/1(Xmt 1)
  Xmt 2/1 -> While Iterator Subsystem/2(Xmt 2)
  While Iterator Subsystem/1(Recv 1) -> Recv 1/1
  While Iterator Subsystem/2(Recv 2) -> Recv 2/1
  Xmt 3/1 -> While Iterator Subsystem/3(Xmt 3)
  Xmt 4/1 -> While Iterator Subsystem/4(Xmt 4)
  While Iterator Subsystem/3(Recv 3) -> Recv 3/1
  While Iterator Subsystem/4(Recv 4) -> Recv 4/1

== system speedgoatlib/IO503/Send Receive/RS232 ISR ==
  Xmt 1 : Inport
  Xmt 2 : Inport  Port=2
  Xmt 3 : Inport  Port=3
  Xmt 4 : Inport  Port=4
  function : TriggerPort  TriggerType=function-call
  While Iterator Subsystem : Subsystem  TreatAsAtomicUnit=on
  Recv 1 : Outport
  Recv 2 : Outport  Port=2
  Recv 3 : Outport  Port=3
  Recv 4 : Outport  Port=4
  wires:
  Xmt 1/1 -> While Iterator Subsystem/1(Xmt 1)
  Xmt 2/1 -> While Iterator Subsystem/2(Xmt 2)
  While Iterator Subsystem/1(Recv 1) -> Recv 1/1
  While Iterator Subsystem/2(Recv 2) -> Recv 2/1
  Xmt 3/1 -> While Iterator Subsystem/3(Xmt 3)
  Xmt 4/1 -> While Iterator Subsystem/4(Xmt 4)
  While Iterator Subsystem/3(Recv 3) -> Recv 3/1
  While Iterator Subsystem/4(Recv 4) -> Recv 4/1

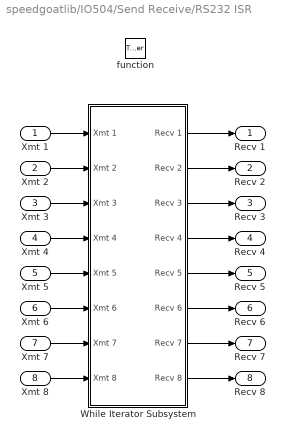
== system speedgoatlib/IO504/Send Receive/RS232 ISR ==
  Xmt 1 : Inport
  Xmt 2 : Inport  Port=2
  Xmt 3 : Inport  Port=3
  Xmt 4 : Inport  Port=4
  Xmt 5 : Inport  Port=5
  Xmt 6 : Inport  Port=6
  Xmt 7 : Inport  Port=7
  Xmt 8 : Inport  Port=8
  function : TriggerPort  TriggerType=function-call
  While Iterator Subsystem : Subsystem  TreatAsAtomicUnit=on
  Recv 1 : Outport
  Recv 2 : Outport  Port=2
  Recv 3 : Outport  Port=3
  Recv 4 : Outport  Port=4
  Recv 5 : Outport  Port=5
  Recv 6 : Outport  Port=6
  Recv 7 : Outport  Port=7
  Recv 8 : Outport  Port=8
  wires:
  While Iterator Subsystem/4(Recv 4) -> Recv 4/1
  While Iterator Subsystem/3(Recv 3) -> Recv 3/1
  Xmt 4/1 -> While Iterator Subsystem/4(Xmt 4)
  Xmt 3/1 -> While Iterator Subsystem/3(Xmt 3)
  While Iterator Subsystem/2(Recv 2) -> Recv 2/1
  While Iterator Subsystem/1(Recv 1) -> Recv 1/1
  Xmt 2/1 -> While Iterator Subsystem/2(Xmt 2)
  Xmt 1/1 -> While Iterator Subsystem/1(Xmt 1)
  Xmt 8/1 -> While Iterator Subsystem/8(Xmt 8)
  Xmt 7/1 -> While Iterator Subsystem/7(Xmt 7)
  Xmt 6/1 -> While Iterator Subsystem/6(Xmt 6)
  Xmt 5/1 -> While Iterator Subsystem/5(Xmt 5)
  While Iterator Subsystem/8(Recv 8) -> Recv 8/1
  While Iterator Subsystem/7(Recv 7) -> Recv 7/1
  While Iterator Subsystem/6(Recv 6) -> Recv 6/1
  While Iterator Subsystem/5(Recv 5) -> Recv 5/1

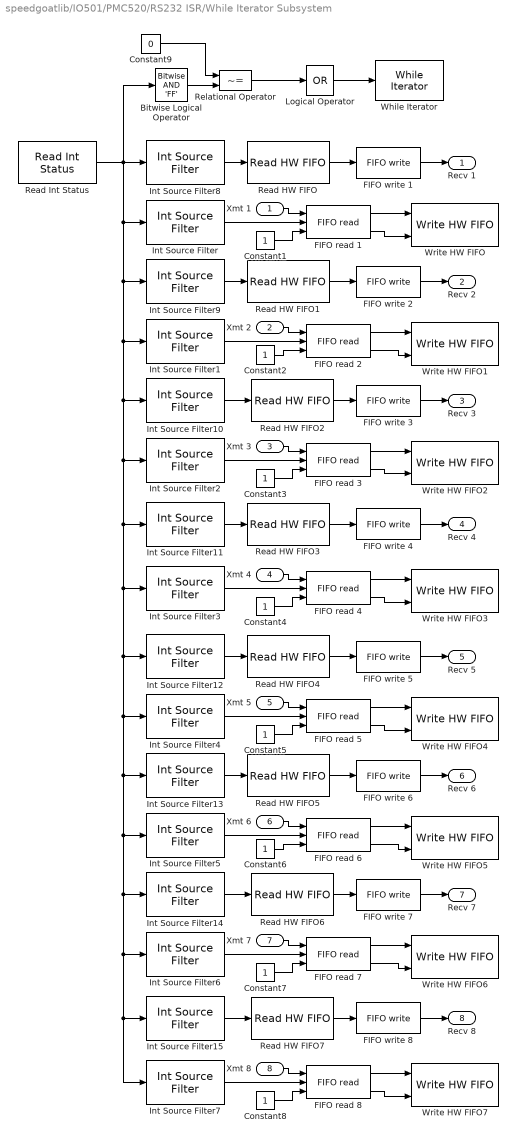
== system speedgoatlib/IO501/PMC520/RS232 ISR/While Iterator Subsystem ==
  Xmt 1 : Inport
  Xmt 2 : Inport  Port=2
  Xmt 3 : Inport  Port=3
  Xmt 4 : Inport  Port=4
  Xmt 5 : Inport  Port=5
  Xmt 6 : Inport  Port=6
  Xmt 7 : Inport  Port=7
  Xmt 8 : Inport  Port=8
  Bitwise Logical Operator : simulink/Logic and Bit Operations/Bitwise Operator  logicop=AND  UseBitMask=on  BitMask='FF'  BitMaskRealWorld=Stored Integer
  Constant{1..8} (8 alike) : Constant  OutDataTypeStr=uint32
  Constant9 : Constant  Value=0  OutDataTypeStr=uint32
  FIFO read {1..8} (8 alike) : xpcseriallib/FIFO read   maxsize=60  minsize=1  usedelimiter=off  delimiter=13  outputtype=count+32 bit uint  enable=on  enableout=on  sampletime=-1
  FIFO write 1 : xpcseriallib/FIFO write   size=1024  inputtype=count+32 bit uint  present=off  sampletime=-1  id=RCV channel 1, IRQ 5
  FIFO write 2 : xpcseriallib/FIFO write   size=1024  inputtype=count+32 bit uint  present=off  sampletime=-1  id=RCV channel 2, IRQ 5
  FIFO write 3 : xpcseriallib/FIFO write   size=1024  inputtype=count+32 bit uint  present=off  sampletime=-1  id=RCV channel 3, IRQ 5
  FIFO write 4 : xpcseriallib/FIFO write   size=1024  inputtype=count+32 bit uint  present=off  sampletime=-1  id=RCV channel 4, IRQ 5
  FIFO write 5 : xpcseriallib/FIFO write   size=1024  inputtype=count+32 bit uint  present=off  sampletime=-1  id=RCV channel 5, IRQ 5
  FIFO write 6 : xpcseriallib/FIFO write   size=1024  inputtype=count+32 bit uint  present=off  sampletime=-1  id=RCV channel 6, IRQ 5
  FIFO write 7 : xpcseriallib/FIFO write   size=1024  inputtype=count+32 bit uint  present=off  sampletime=-1  id=RCV channel 7, IRQ 5
  FIFO write 8 : xpcseriallib/FIFO write   size=1024  inputtype=count+32 bit uint  present=off  sampletime=-1  id=RCV channel 8, IRQ 5
  Int Source Filter : speedgoatlib/IO501/Acromag PMC520 Internal blocks/Int Source Filter  port=1  value=Transmitter empty
  Int Source Filter1 : speedgoatlib/IO501/Acromag PMC520 Internal blocks/Int Source Filter  port=2  value=Transmitter empty
  Int Source Filter10 : speedgoatlib/IO501/Acromag PMC520 Internal blocks/Int Source Filter  port=3  value=Receive data
  Int Source Filter11 : speedgoatlib/IO501/Acromag PMC520 Internal blocks/Int Source Filter  port=4  value=Receive data
  Int Source Filter12 : speedgoatlib/IO501/Acromag PMC520 Internal blocks/Int Source Filter  port=5  value=Receive data
  Int Source Filter13 : speedgoatlib/IO501/Acromag PMC520 Internal blocks/Int Source Filter  port=6  value=Receive data
  Int Source Filter14 : speedgoatlib/IO501/Acromag PMC520 Internal blocks/Int Source Filter  port=7  value=Receive data
  Int Source Filter15 : speedgoatlib/IO501/Acromag PMC520 Internal blocks/Int Source Filter  port=8  value=Receive data
  Int Source Filter2 : speedgoatlib/IO501/Acromag PMC520 Internal blocks/Int Source Filter  port=3  value=Transmitter empty
  Int Source Filter3 : speedgoatlib/IO501/Acromag PMC520 Internal blocks/Int Source Filter  port=4  value=Transmitter empty
  Int Source Filter4 : speedgoatlib/IO501/Acromag PMC520 Internal blocks/Int Source Filter  port=5  value=Transmitter empty
  Int Source Filter5 : speedgoatlib/IO501/Acromag PMC520 Internal blocks/Int Source Filter  port=6  value=Transmitter empty
  Int Source Filter6 : speedgoatlib/IO501/Acromag PMC520 Internal blocks/Int Source Filter  port=7  value=Transmitter empty
  Int Source Filter7 : speedgoatlib/IO501/Acromag PMC520 Internal blocks/Int Source Filter  port=8  value=Transmitter empty
  Int Source Filter8 : speedgoatlib/IO501/Acromag PMC520 Internal blocks/Int Source Filter  port=1  value=Receive data
  Int Source Filter9 : speedgoatlib/IO501/Acromag PMC520 Internal blocks/Int Source Filter  port=2  value=Receive data
  Logical Operator : Logic  Operator=OR  Inputs=1  AllPortsSameDT=off
  Read HW FIFO : speedgoatlib/IO501/Acromag PMC520 Internal blocks/Read HW FIFO  port=1  flush=on  slot=subslot
  Read HW FIFO1 : speedgoatlib/IO501/Acromag PMC520 Internal blocks/Read HW FIFO  port=2  flush=on  slot=subslot
  Read HW FIFO2 : speedgoatlib/IO501/Acromag PMC520 Internal blocks/Read HW FIFO  port=3  flush=on  slot=subslot
  Read HW FIFO3 : speedgoatlib/IO501/Acromag PMC520 Internal blocks/Read HW FIFO  port=4  flush=on  slot=subslot
  Read HW FIFO4 : speedgoatlib/IO501/Acromag PMC520 Internal blocks/Read HW FIFO  port=5  flush=on  slot=subslot
  Read HW FIFO5 : speedgoatlib/IO501/Acromag PMC520 Internal blocks/Read HW FIFO  port=6  flush=on  slot=subslot
  Read HW FIFO6 : speedgoatlib/IO501/Acromag PMC520 Internal blocks/Read HW FIFO  port=7  flush=on  slot=subslot
  Read HW FIFO7 : speedgoatlib/IO501/Acromag PMC520 Internal blocks/Read HW FIFO  port=8  flush=on  slot=subslot
  Read Int Status : speedgoatlib/IO501/Acromag PMC520 Internal blocks/Read Int Status  slot=subslot
  Relational Operator : RelationalOperator  Operator=~=
  While Iterator : WhileIterator  MaxIters=65  WhileBlockType=do-while
  Write HW FIFO : speedgoatlib/IO501/Acromag PMC520 Internal blocks/Write HW FIFO  port=1  slot=subslot
  Write HW FIFO1 : speedgoatlib/IO501/Acromag PMC520 Internal blocks/Write HW FIFO  port=2  slot=subslot
  Write HW FIFO2 : speedgoatlib/IO501/Acromag PMC520 Internal blocks/Write HW FIFO  port=3  slot=subslot
  Write HW FIFO3 : speedgoatlib/IO501/Acromag PMC520 Internal blocks/Write HW FIFO  port=4  slot=subslot
  Write HW FIFO4 : speedgoatlib/IO501/Acromag PMC520 Internal blocks/Write HW FIFO  port=5  slot=subslot
  Write HW FIFO5 : speedgoatlib/IO501/Acromag PMC520 Internal blocks/Write HW FIFO  port=6  slot=subslot
  Write HW FIFO6 : speedgoatlib/IO501/Acromag PMC520 Internal blocks/Write HW FIFO  port=7  slot=subslot
  Write HW FIFO7 : speedgoatlib/IO501/Acromag PMC520 Internal blocks/Write HW FIFO  port=8  slot=subslot
  Recv 1 : Outport
  Recv 2 : Outport  Port=2
  Recv 3 : Outport  Port=3
  Recv 4 : Outport  Port=4
  Recv 5 : Outport  Port=5
  Recv 6 : Outport  Port=6
  Recv 7 : Outport  Port=7
  Recv 8 : Outport  Port=8
  wires:
  Read HW FIFO3/1 -> FIFO write 4/1
  FIFO write 4/1 -> Recv 4/1
  Read HW FIFO2/1 -> FIFO write 3/1
  FIFO write 3/1 -> Recv 3/1
  Int Source Filter11/1 -> Read HW FIFO3/1
  Int Source Filter10/1 -> Read HW FIFO2/1
  Constant4/1 -> FIFO read 4/3
  FIFO read 4/2 -> Write HW FIFO3/2
  FIFO read 4/1 -> Write HW FIFO3/1
  Xmt 4/1 -> FIFO read 4/1
  Int Source Filter3/1 -> FIFO read 4/2
  Constant3/1 -> FIFO read 3/3
  FIFO read 3/2 -> Write HW FIFO2/2
  FIFO read 3/1 -> Write HW FIFO2/1
  Xmt 3/1 -> FIFO read 3/1
  Int Source Filter2/1 -> FIFO read 3/2
  Constant2/1 -> FIFO read 2/3
  Constant1/1 -> FIFO read 1/3
  FIFO read 2/2 -> Write HW FIFO1/2
  FIFO read 1/2 -> Write HW FIFO/2
  FIFO read 1/1 -> Write HW FIFO/1
  FIFO read 2/1 -> Write HW FIFO1/1
  Xmt 2/1 -> FIFO read 2/1
  Int Source Filter1/1 -> FIFO read 2/2
  Read HW FIFO1/1 -> FIFO write 2/1
  FIFO write 2/1 -> Recv 2/1
  Int Source Filter9/1 -> Read HW FIFO1/1
  Xmt 1/1 -> FIFO read 1/1
  Int Source Filter/1 -> FIFO read 1/2
  Read HW FIFO/1 -> FIFO write 1/1
  FIFO write 1/1 -> Recv 1/1
  Int Source Filter8/1 -> Read HW FIFO/1
  Read Int Status/1 -> Bitwise Logical Operator/1, Int Source Filter15/1, Int Source Filter7/1, Int Source Filter6/1, Int Source Filter14/1, Int Source Filter5/1, Int Source Filter13/1, Int Source Filter4/1, Int Source Filter12/1, Int Source Filter3/1, Int Source Filter11/1, Int Source Filter2/1, Int Source Filter10/1, Int Source Filter1/1, Int Source Filter9/1, Int Source Filter/1, Int Source Filter8/1
  Constant9/1 -> Relational Operator/1
  Bitwise Logical Operator/1 -> Relational Operator/2
  Relational Operator/1 -> Logical Operator/1
  Logical Operator/1 -> While Iterator/1
  Read HW FIFO7/1 -> FIFO write 8/1
  FIFO write 8/1 -> Recv 8/1
  Read HW FIFO6/1 -> FIFO write 7/1
  FIFO write 7/1 -> Recv 7/1
  Int Source Filter15/1 -> Read HW FIFO7/1
  Int Source Filter14/1 -> Read HW FIFO6/1
  Constant8/1 -> FIFO read 8/3
  FIFO read 8/2 -> Write HW FIFO7/2
  FIFO read 8/1 -> Write HW FIFO7/1
  Xmt 8/1 -> FIFO read 8/1
  Int Source Filter7/1 -> FIFO read 8/2
  Constant7/1 -> FIFO read 7/3
  FIFO read 7/2 -> Write HW FIFO6/2
  FIFO read 7/1 -> Write HW FIFO6/1
  Xmt 7/1 -> FIFO read 7/1
  Int Source Filter6/1 -> FIFO read 7/2
  Constant6/1 -> FIFO read 6/3
  Constant5/1 -> FIFO read 5/3
  FIFO read 6/2 -> Write HW FIFO5/2
  FIFO read 5/2 -> Write HW FIFO4/2
  FIFO read 5/1 -> Write HW FIFO4/1
  FIFO read 6/1 -> Write HW FIFO5/1
  Xmt 6/1 -> FIFO read 6/1
  Int Source Filter5/1 -> FIFO read 6/2
  Read HW FIFO5/1 -> FIFO write 6/1
  FIFO write 6/1 -> Recv 6/1
  Int Source Filter13/1 -> Read HW FIFO5/1
  Xmt 5/1 -> FIFO read 5/1
  Int Source Filter4/1 -> FIFO read 5/2
  Read HW FIFO4/1 -> FIFO write 5/1
  FIFO write 5/1 -> Recv 5/1
  Int Source Filter12/1 -> Read HW FIFO4/1
